simulink model "model_local_observers"  (R2024b)
settings: Solver=ode45  StartTime=0.0  StopTime=150  RelTol=1e-3
values from neighbouring files (symbols this model uses):
  Ad = [ ... (first row only)    [compute_topology_matrices.m]
  G = diag([1 1 1 1 1 1])    [compute_topology_matrices.m]
undefined symbols (not defined in the file or in its folder): A, A_leader, B, C, c, F, K, Lu_obs, noise_free, sigma_followers, sigma_leader, x0, x0_followers, xhat0
settings Model: Creator=siani  LastModifiedBy=siani
settings DebuggingCC: AlgebraicLoopMsg=none

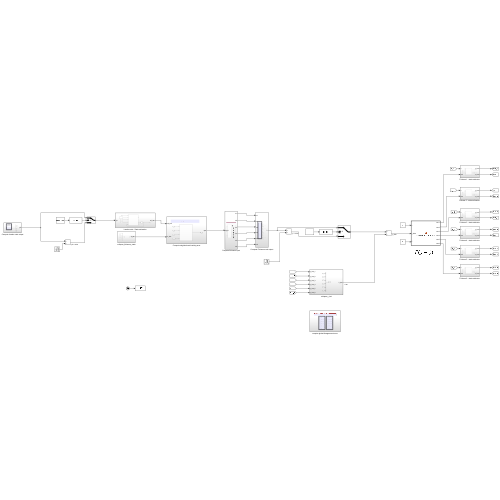
[thumbnail: Simulink's stored preview of the top-level diagram]
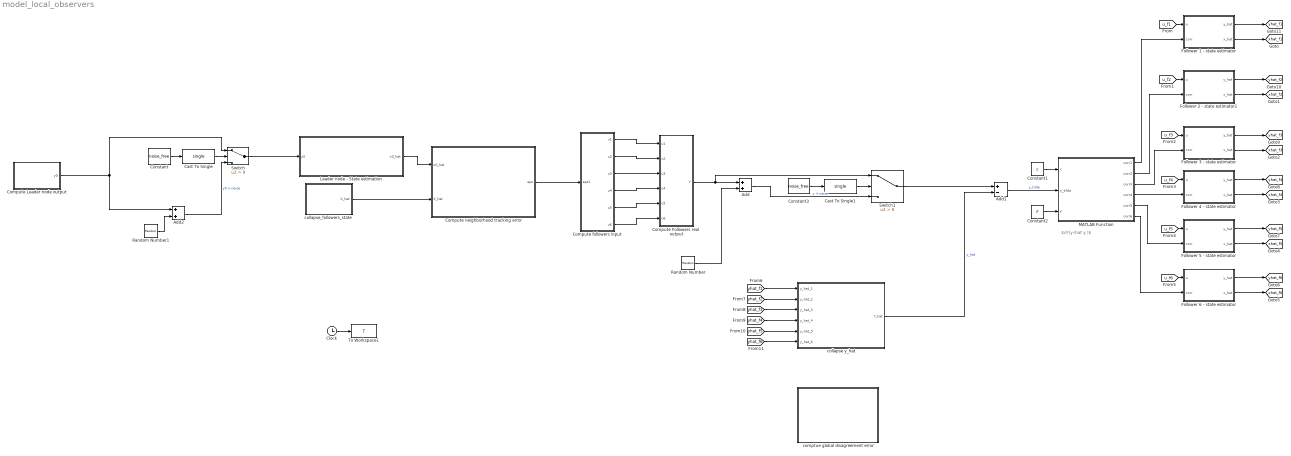
== system model_local_observers ==
  note: $cF(y-\hat y )$
  Add : Sum
  Add1 : Sum  Inputs=+-
  Add2 : Sum
  Cast To Single : DataTypeConversion  OutDataTypeStr=single  SaturateOnIntegerOverflow=off  RndMeth=Floor
  Cast To Single1 : DataTypeConversion  OutDataTypeStr=single  SaturateOnIntegerOverflow=off  RndMeth=Floor
  Clock : Clock
  Compute Followers real output : Subsystem
  Compute Leader node output : Subsystem
  Compute followers input : Subsystem
  Compute neighborhood tracking error : Subsystem
  Constant : Constant  Value=noise_free
  Constant1 : Constant  Value=c
  Constant2 : Constant  Value=F
  Constant3 : Constant  Value=noise_free
  Follower 1 - state estimator : Subsystem
  Follower 2 - state estimator1 : Subsystem
  Follower 3 - state estimator : Subsystem
  Follower 4 - state estimator : Subsystem
  Follower 5 - state estimator : Subsystem
  Follower 6 - state estimator : Subsystem
  Leader node - State estimation : Subsystem
  MATLAB Function : MATLAB Function  TreatAsAtomicUnit=on
  Random Number : RandomNumber  Mean=zeros(6,1)  Variance=sigma_followers^2*ones(6,1)  SampleTime=0.1
  Random Number1 : RandomNumber  Variance=sigma_leader^2  SampleTime=0.1
  Switch : Switch  Criteria=u2 > Threshold  SaturateOnIntegerOverflow=off  InputSameDT=off
  Switch1 : Switch  Criteria=u2 > Threshold  SaturateOnIntegerOverflow=off  InputSameDT=off
  To Workspace1 : ToWorkspace  VariableName=T  SampleTime=-1
  collapse y_hat : Subsystem
  collapse_followers_state : Subsystem
  comptue global disagreement error : Subsystem
  tag scope: xhat_f1=global, xhat_f2=global, xhat_f3=global, xhat_f4=global, xhat_f5=global, xhat_f6=global, yhat_f1=global, yhat_f2=global, yhat_f3=global, yhat_f4=global, yhat_f5=global, yhat_f6=global
  wires:
  Compute Followers real output/1(Y) -> Switch1/1, Add/1
  [u_f1] -> Follower 1 - state estimator/1(u)
  Switch/1 -> Leader node - State estimation/1(y0)
  Switch1/1 -> Add1/1
  Add/1 -> Switch1/3  "y + noise"
  Compute Leader node output/1(y0) -> Add2/1, Switch/1
  collapse y_hat/1(Y_hat) -> Add1/2  "y_hat"
  Add1/1 -> MATLAB Function/2(y_tilda)  "y_tilda"
  [yhat_f1] -> collapse y_hat/1(y_hat_1)
  [yhat_f2] -> collapse y_hat/2(y_hat_2)
  [yhat_f3] -> collapse y_hat/3(y_hat_3)
  [yhat_f4] -> collapse y_hat/4(y_hat_4)
  [yhat_f5] -> collapse y_hat/5(y_hat_5)
  [yhat_f6] -> collapse y_hat/6(y_hat_6)
  Random Number/1 -> Add/2
  Leader node - State estimation/1(x0_hat) -> Compute neighborhood tracking error/1(x0_hat)
  collapse_followers_state/1(X_hat) -> Compute neighborhood tracking error/2(X_hat)
  Constant1/1 -> MATLAB Function/1(c)
  Constant2/1 -> MATLAB Function/3(F)
  MATLAB Function/1(corr1) -> Follower 1 - state estimator/2(corr)
  MATLAB Function/2(corr2) -> Follower 2 - state estimator1/2(corr)
  MATLAB Function/3(corr3) -> Follower 3 - state estimator/2(corr)
  MATLAB Function/4(corr4) -> Follower 4 - state estimator/2(corr)
  MATLAB Function/5(corr5) -> Follower 5 - state estimator/2(corr)
  MATLAB Function/6(corr6) -> Follower 6 - state estimator/2(corr)
  Follower 1 - state estimator/1(y_hat) -> [yhat_f1]
  Follower 1 - state estimator/2(x_hat) -> [xhat_f1]
  Follower 2 - state estimator1/1(y_hat) -> [yhat_f2]
  Follower 2 - state estimator1/2(x_hat) -> [xhat_f2]
  Follower 3 - state estimator/1(y_hat) -> [yhat_f3]
  Follower 3 - state estimator/2(x_hat) -> [xhat_f3]
  Follower 4 - state estimator/1(y_hat) -> [yhat_f4]
  Follower 4 - state estimator/2(x_hat) -> [xhat_f4]
  Follower 5 - state estimator/1(y_hat) -> [yhat_f5]
  Follower 5 - state estimator/2(x_hat) -> [xhat_f5]
  Follower 6 - state estimator/1(y_hat) -> [yhat_f6]
  Follower 6 - state estimator/2(x_hat) -> [xhat_f6]
  [u_f2] -> Follower 2 - state estimator1/1(u)
  [u_f3] -> Follower 3 - state estimator/1(u)
  [u_f4] -> Follower 4 - state estimator/1(u)
  [u_f5] -> Follower 5 - state estimator/1(u)
  [u_f6] -> Follower 6 - state estimator/1(u)
  Constant3/1 -> Cast To Single1/1
  Cast To Single1/1 -> Switch1/2
  Add2/1 -> Switch/3  "y0 + noise"
  Cast To Single/1 -> Switch/2
  Constant/1 -> Cast To Single/1
  Random Number1/1 -> Add2/2
  Clock/1 -> To Workspace1/1
  Compute neighborhood tracking error/1(eps) -> Compute followers input/1(eps1)
  Compute followers input/1(u1) -> Compute Followers real output/1(u1)
  Compute followers input/2(u2) -> Compute Followers real output/2(u2)
  Compute followers input/3(u3) -> Compute Followers real output/3(u3)
  Compute followers input/4(u4) -> Compute Followers real output/4(u4)
  Compute followers input/5(u5) -> Compute Followers real output/5(u5)
  Compute followers input/6(u6) -> Compute Followers real output/6(u6)

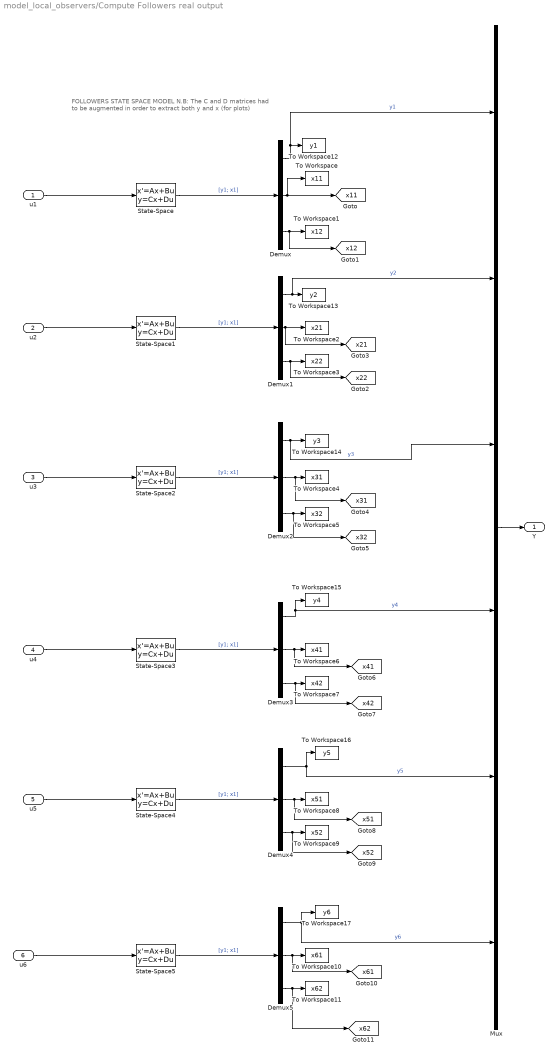
== system model_local_observers/Compute Followers real output ==
  note: FOLLOWERS STATE SPACE MODEL
      |
      | N.B: The C and D matrices had to be augmented in order to extract both y and x (for plots)
  u1 : Inport
  u2 : Inport  Port=2
  u3 : Inport  Port=3
  u4 : Inport  Port=4
  u5 : Inport  Port=5
  u6 : Inport  Port=6
  Demux{,1..5} (6 alike) : Demux  Outputs=[1 1 1]
  Mux : Mux  Inputs=[1 1 1 1 1 1]
  State-Space{,1..5} (6 alike) : StateSpace  A=A  B=B  C=[C;eye(2)]  D=[0;0;0]  InitialCondition=x0_followers
  To Workspace : ToWorkspace  VariableName=x11  SampleTime=-1
  To Workspace1 : ToWorkspace  VariableName=x12  SampleTime=-1
  To Workspace10 : ToWorkspace  VariableName=x61  SampleTime=-1
  To Workspace11 : ToWorkspace  VariableName=x62  SampleTime=-1
  To Workspace12 : ToWorkspace  VariableName=y1  SampleTime=-1
  To Workspace13 : ToWorkspace  VariableName=y2  SampleTime=-1
  To Workspace14 : ToWorkspace  VariableName=y3  SampleTime=-1
  To Workspace15 : ToWorkspace  VariableName=y4  SampleTime=-1
  To Workspace16 : ToWorkspace  VariableName=y5  SampleTime=-1
  To Workspace17 : ToWorkspace  VariableName=y6  SampleTime=-1
  To Workspace2 : ToWorkspace  VariableName=x21  SampleTime=-1
  To Workspace3 : ToWorkspace  VariableName=x22  SampleTime=-1
  To Workspace4 : ToWorkspace  VariableName=x31  SampleTime=-1
  To Workspace5 : ToWorkspace  VariableName=x32  SampleTime=-1
  To Workspace6 : ToWorkspace  VariableName=x41  SampleTime=-1
  To Workspace7 : ToWorkspace  VariableName=x42  SampleTime=-1
  To Workspace8 : ToWorkspace  VariableName=x51  SampleTime=-1
  To Workspace9 : ToWorkspace  VariableName=x52  SampleTime=-1
  Y : Outport
  tag scope: x11=global, x12=global, x21=global, x22=global, x31=global, x32=global, x41=global, x42=global, x51=global, x52=global, x61=global, x62=global
  wires:
  u1/1 -> State-Space/1
  Mux/1 -> Y/1
  State-Space/1 -> Demux/1  "[y1; x1]"
  Demux/1 -> To Workspace12/1, Mux/1  "y1"
  Demux/2 -> To Workspace/1, [x11]
  Demux/3 -> [x12], To Workspace1/1
  Demux1/2 -> [x21], To Workspace2/1
  State-Space1/1 -> Demux1/1  "[y1; x1]"
  Demux1/3 -> [x22], To Workspace3/1
  Demux1/1 -> Mux/2, To Workspace13/1  "y2"
  u2/1 -> State-Space1/1
  Demux2/1 -> Mux/3, To Workspace14/1  "y3"
  Demux2/3 -> [x32], To Workspace5/1
  Demux2/2 -> [x31], To Workspace4/1
  State-Space2/1 -> Demux2/1  "[y1; x1]"
  u3/1 -> State-Space2/1
  Demux3/2 -> [x41], To Workspace6/1
  Demux3/3 -> [x42], To Workspace7/1
  State-Space3/1 -> Demux3/1  "[y1; x1]"
  Demux3/1 -> To Workspace15/1, Mux/4  "y4"
  u4/1 -> State-Space3/1
  Demux4/3 -> [x52], To Workspace9/1
  Demux4/2 -> [x51], To Workspace8/1
  State-Space4/1 -> Demux4/1  "[y1; x1]"
  u5/1 -> State-Space4/1
  State-Space5/1 -> Demux5/1  "[y1; x1]"
  Demux5/2 -> [x61], To Workspace10/1
  Demux5/3 -> [x62], To Workspace11/1
  u6/1 -> State-Space5/1
  Demux4/1 -> Mux/5, To Workspace16/1  "y5"
  Demux5/1 -> Mux/6, To Workspace17/1  "y6"

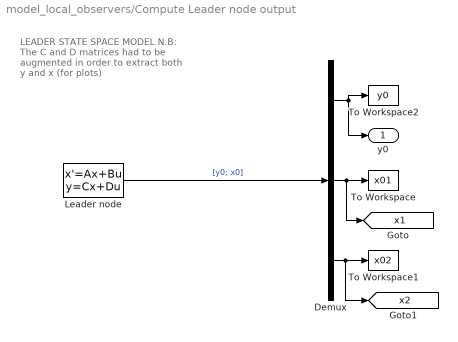
== system model_local_observers/Compute Leader node output ==
  note: LEADER STATE SPACE MODEL
      |
      | N.B: The C and D matrices had to be augmented in order to extract both y and x (for plots)
  Demux : Demux  Outputs=[1 1 1]
  Leader node : StateSpace  A=A_leader  B=[0 0]'  C=[C;eye(2)]  D=[0;0;0]  InitialCondition=x0
  To Workspace : ToWorkspace  VariableName=x01  SampleTime=-1
  To Workspace1 : ToWorkspace  VariableName=x02  SampleTime=-1
  To Workspace2 : ToWorkspace  VariableName=y0  SampleTime=-1
  y0 : Outport
  tag scope: x1=global, x2=global
  wires:
  Leader node/1 -> Demux/1  "[y0; x0]"
  Demux/1 -> To Workspace2/1, y0/1
  Demux/2 -> [x1], To Workspace/1
  Demux/3 -> [x2], To Workspace1/1

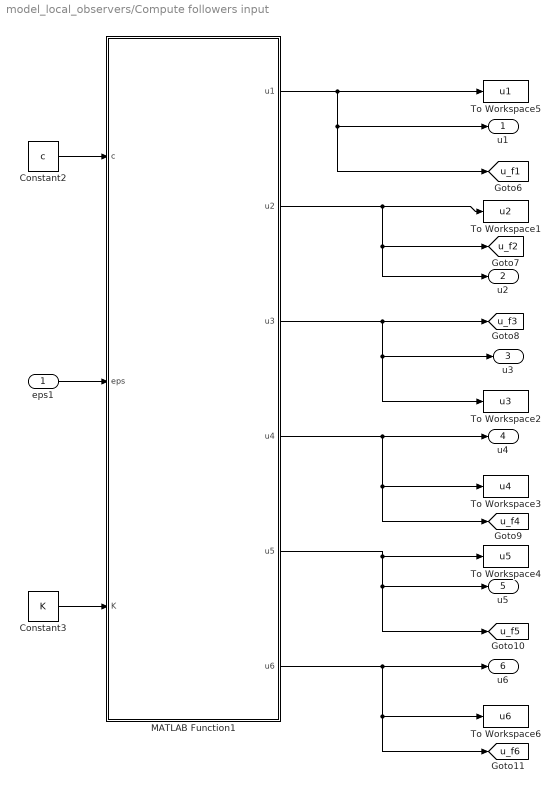
== system model_local_observers/Compute followers input ==
  eps1 : Inport
  Constant2 : Constant  Value=c
  Constant3 : Constant  Value=K  VectorParams1D=off
  MATLAB Function1 : MATLAB Function  TreatAsAtomicUnit=on
  To Workspace1 : ToWorkspace  VariableName=u2  SampleTime=-1
  To Workspace2 : ToWorkspace  VariableName=u3  SampleTime=-1
  To Workspace3 : ToWorkspace  VariableName=u4  SampleTime=-1
  To Workspace4 : ToWorkspace  VariableName=u5  SampleTime=-1
  To Workspace5 : ToWorkspace  VariableName=u1  SampleTime=-1
  To Workspace6 : ToWorkspace  VariableName=u6  SampleTime=-1
  u1 : Outport
  u2 : Outport  Port=2
  u3 : Outport  Port=3
  u4 : Outport  Port=4
  u5 : Outport  Port=5
  u6 : Outport  Port=6
  tag scope: u_f1=global, u_f2=global, u_f3=global, u_f4=global, u_f5=global, u_f6=global
  wires:
  MATLAB Function1/3(u3) -> u3/1, To Workspace2/1, [u_f3]
  MATLAB Function1/5(u5) -> u5/1, [u_f5], To Workspace4/1
  MATLAB Function1/6(u6) -> [u_f6], To Workspace6/1, u6/1
  eps1/1 -> MATLAB Function1/2(eps)
  MATLAB Function1/4(u4) -> [u_f4], To Workspace3/1, u4/1
  Constant2/1 -> MATLAB Function1/1(c)
  Constant3/1 -> MATLAB Function1/3(K)
  MATLAB Function1/2(u2) -> u2/1, [u_f2], To Workspace1/1
  MATLAB Function1/1(u1) -> u1/1, [u_f1], To Workspace5/1

== system model_local_observers/Compute neighborhood tracking error ==
  x0_hat : Inport
  X_hat : Inport  Port=2
  Constant : Constant  Value=Ad
  Constant1 : Constant  Value=G
  MATLAB Function : MATLAB Function  TreatAsAtomicUnit=on
  eps : Outport
  wires:
  x0_hat/1 -> MATLAB Function/2(x0_hat)
  Constant/1 -> MATLAB Function/3(Ad)
  Constant1/1 -> MATLAB Function/4(G)
  X_hat/1 -> MATLAB Function/1(x_hat)
  MATLAB Function/1(eps) -> eps/1

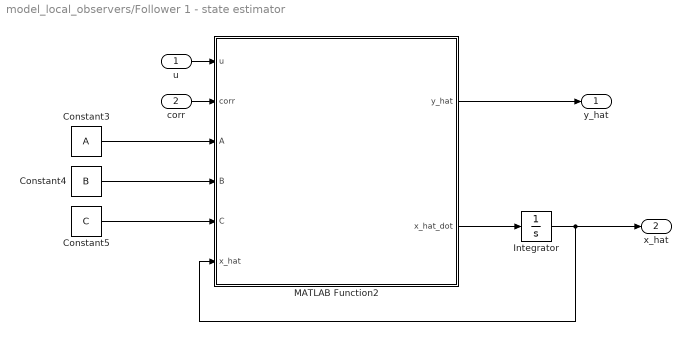
== system model_local_observers/Follower 1 - state estimator ==
  u : Inport
  corr : Inport  Port=2
  Constant3 : Constant  Value=A
  Constant4 : Constant  Value=B  VectorParams1D=off
  Constant5 : Constant  Value=C  VectorParams1D=off
  Integrator : Integrator  InitialCondition=xhat0
  MATLAB Function2 : MATLAB Function  TreatAsAtomicUnit=on
  y_hat : Outport
  x_hat : Outport  Port=2
  wires:
  MATLAB Function2/1(y_hat) -> y_hat/1
  corr/1 -> MATLAB Function2/2(corr)
  MATLAB Function2/2(x_hat_dot) -> Integrator/1
  Integrator/1 -> MATLAB Function2/6(x_hat), x_hat/1
  Constant3/1 -> MATLAB Function2/3(A)
  u/1 -> MATLAB Function2/1(u)
  Constant4/1 -> MATLAB Function2/4(B)
  Constant5/1 -> MATLAB Function2/5(C)

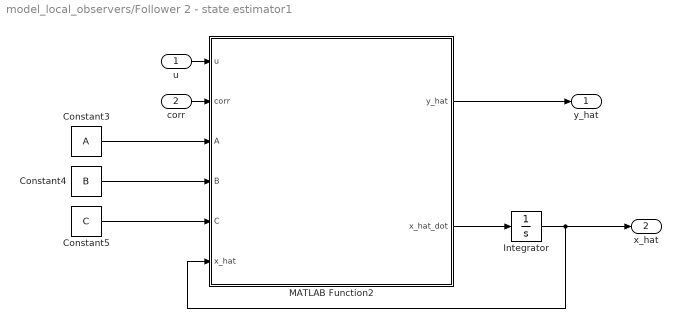
== system model_local_observers/Follower 2 - state estimator1 ==
  u : Inport
  corr : Inport  Port=2
  Constant3 : Constant  Value=A
  Constant4 : Constant  Value=B  VectorParams1D=off
  Constant5 : Constant  Value=C  VectorParams1D=off
  Integrator : Integrator  InitialCondition=xhat0
  MATLAB Function2 : MATLAB Function  TreatAsAtomicUnit=on
  y_hat : Outport
  x_hat : Outport  Port=2
  wires:
  Constant5/1 -> MATLAB Function2/5(C)
  Constant4/1 -> MATLAB Function2/4(B)
  u/1 -> MATLAB Function2/1(u)
  Constant3/1 -> MATLAB Function2/3(A)
  Integrator/1 -> MATLAB Function2/6(x_hat), x_hat/1
  MATLAB Function2/2(x_hat_dot) -> Integrator/1
  corr/1 -> MATLAB Function2/2(corr)
  MATLAB Function2/1(y_hat) -> y_hat/1

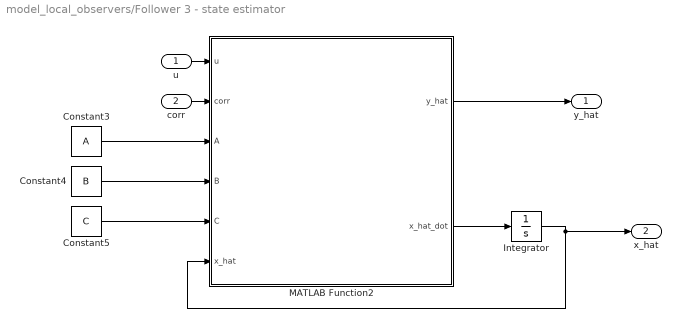
== system model_local_observers/Follower 3 - state estimator ==
  u : Inport
  corr : Inport  Port=2
  Constant3 : Constant  Value=A
  Constant4 : Constant  Value=B  VectorParams1D=off
  Constant5 : Constant  Value=C  VectorParams1D=off
  Integrator : Integrator  InitialCondition=xhat0
  MATLAB Function2 : MATLAB Function  TreatAsAtomicUnit=on
  y_hat : Outport
  x_hat : Outport  Port=2
  wires:
  MATLAB Function2/1(y_hat) -> y_hat/1
  corr/1 -> MATLAB Function2/2(corr)
  MATLAB Function2/2(x_hat_dot) -> Integrator/1
  Integrator/1 -> MATLAB Function2/6(x_hat), x_hat/1
  Constant3/1 -> MATLAB Function2/3(A)
  u/1 -> MATLAB Function2/1(u)
  Constant4/1 -> MATLAB Function2/4(B)
  Constant5/1 -> MATLAB Function2/5(C)

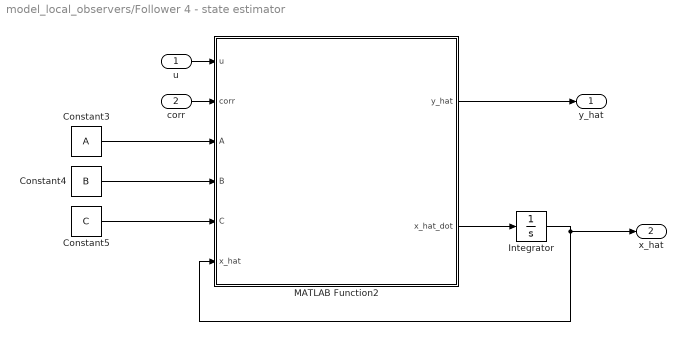
== system model_local_observers/Follower 4 - state estimator ==
  u : Inport
  corr : Inport  Port=2
  Constant3 : Constant  Value=A
  Constant4 : Constant  Value=B  VectorParams1D=off
  Constant5 : Constant  Value=C  VectorParams1D=off
  Integrator : Integrator  InitialCondition=xhat0
  MATLAB Function2 : MATLAB Function  TreatAsAtomicUnit=on
  y_hat : Outport
  x_hat : Outport  Port=2
  wires:
  Constant5/1 -> MATLAB Function2/5(C)
  Constant4/1 -> MATLAB Function2/4(B)
  u/1 -> MATLAB Function2/1(u)
  Constant3/1 -> MATLAB Function2/3(A)
  Integrator/1 -> MATLAB Function2/6(x_hat), x_hat/1
  MATLAB Function2/2(x_hat_dot) -> Integrator/1
  corr/1 -> MATLAB Function2/2(corr)
  MATLAB Function2/1(y_hat) -> y_hat/1

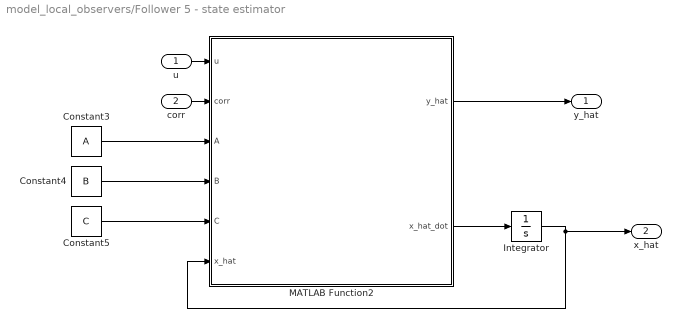
== system model_local_observers/Follower 5 - state estimator ==
  u : Inport
  corr : Inport  Port=2
  Constant3 : Constant  Value=A
  Constant4 : Constant  Value=B  VectorParams1D=off
  Constant5 : Constant  Value=C  VectorParams1D=off
  Integrator : Integrator  InitialCondition=xhat0
  MATLAB Function2 : MATLAB Function  TreatAsAtomicUnit=on
  y_hat : Outport
  x_hat : Outport  Port=2
  wires:
  MATLAB Function2/1(y_hat) -> y_hat/1
  corr/1 -> MATLAB Function2/2(corr)
  MATLAB Function2/2(x_hat_dot) -> Integrator/1
  Integrator/1 -> MATLAB Function2/6(x_hat), x_hat/1
  Constant3/1 -> MATLAB Function2/3(A)
  u/1 -> MATLAB Function2/1(u)
  Constant4/1 -> MATLAB Function2/4(B)
  Constant5/1 -> MATLAB Function2/5(C)

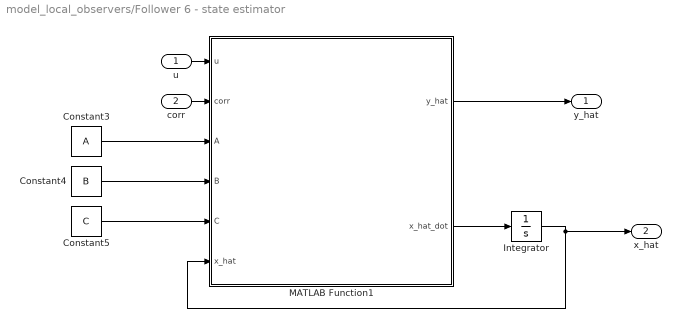
== system model_local_observers/Follower 6 - state estimator ==
  u : Inport
  corr : Inport  Port=2
  Constant3 : Constant  Value=A
  Constant4 : Constant  Value=B  VectorParams1D=off
  Constant5 : Constant  Value=C  VectorParams1D=off
  Integrator : Integrator  InitialCondition=xhat0
  MATLAB Function1 : MATLAB Function  TreatAsAtomicUnit=on
  y_hat : Outport
  x_hat : Outport  Port=2
  wires:
  Constant5/1 -> MATLAB Function1/5(C)
  Constant4/1 -> MATLAB Function1/4(B)
  u/1 -> MATLAB Function1/1(u)
  Constant3/1 -> MATLAB Function1/3(A)
  Integrator/1 -> MATLAB Function1/6(x_hat), x_hat/1
  MATLAB Function1/2(x_hat_dot) -> Integrator/1
  corr/1 -> MATLAB Function1/2(corr)
  MATLAB Function1/1(y_hat) -> y_hat/1

== system model_local_observers/Leader node - State estimation ==
  y0 : Inport
  Constant3 : Constant  Value=A_leader
  Constant4 : Constant  Value=Lu_obs  VectorParams1D=off
  Constant5 : Constant  Value=C  VectorParams1D=off
  Integrator : Integrator  InitialCondition=xhat0
  MATLAB Function1 : MATLAB Function  TreatAsAtomicUnit=on
  x0_hat : Outport
  wires:
  Constant3/1 -> MATLAB Function1/2(A)
  Integrator/1 -> MATLAB Function1/5(x0_hat), x0_hat/1
  Constant5/1 -> MATLAB Function1/3(C)
  Constant4/1 -> MATLAB Function1/4(L)
  MATLAB Function1/2(x0_hat_dot) -> Integrator/1
  y0/1 -> MATLAB Function1/1(y0)

== system model_local_observers/collapse y_hat ==
  y_hat_1 : Inport
  y_hat_2 : Inport  Port=2
  y_hat_3 : Inport  Port=3
  y_hat_4 : Inport  Port=4
  y_hat_5 : Inport  Port=5
  y_hat_6 : Inport  Port=6
  Mux : Mux  Inputs=6
  Y_hat : Outport
  wires:
  y_hat_1/1 -> Mux/1
  Mux/1 -> Y_hat/1
  y_hat_4/1 -> Mux/4
  y_hat_3/1 -> Mux/3
  y_hat_6/1 -> Mux/6
  y_hat_2/1 -> Mux/2
  y_hat_5/1 -> Mux/5

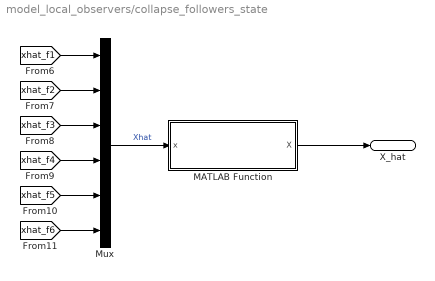
== system model_local_observers/collapse_followers_state ==
  MATLAB Function : MATLAB Function  TreatAsAtomicUnit=on
  Mux : Mux  Inputs=[2 2 2 2 2 2 ]
  X_hat : Outport
  wires:
  [xhat_f2] -> Mux/2
  [xhat_f5] -> Mux/5
  [xhat_f6] -> Mux/6
  [xhat_f3] -> Mux/3
  [xhat_f4] -> Mux/4
  [xhat_f1] -> Mux/1
  MATLAB Function/1(X) -> X_hat/1
  Mux/1 -> MATLAB Function/1(x)  "Xhat"

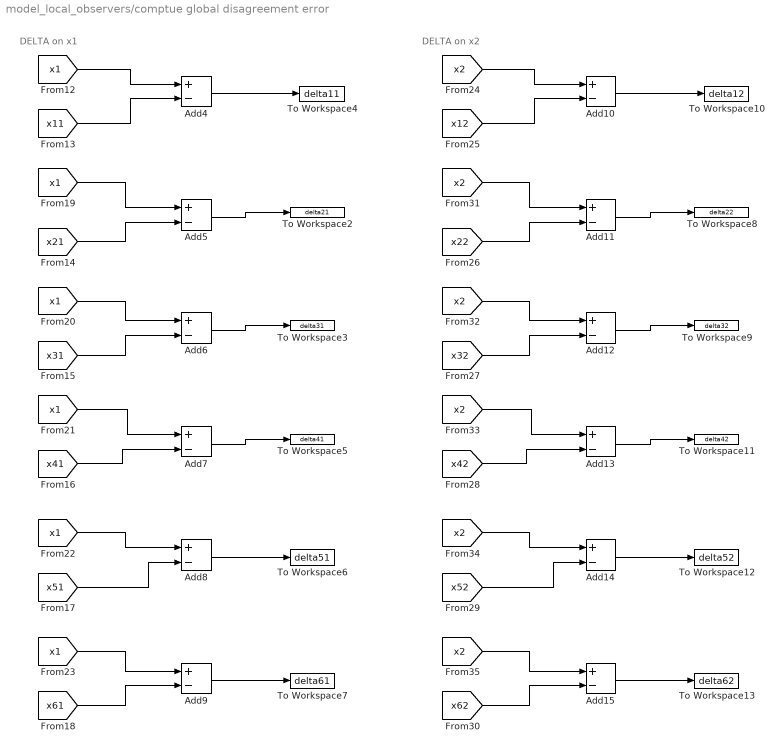
== system model_local_observers/comptue global disagreement error ==
  note: DELTA on x2
  note: DELTA on x1
  Add{4..15} (12 alike) : Sum  Inputs=+-
  To Workspace10 : ToWorkspace  VariableName=delta12  SampleTime=-1
  To Workspace11 : ToWorkspace  VariableName=delta42  SampleTime=-1
  To Workspace12 : ToWorkspace  VariableName=delta52  SampleTime=-1
  To Workspace13 : ToWorkspace  VariableName=delta62  SampleTime=-1
  To Workspace2 : ToWorkspace  VariableName=delta21  SampleTime=-1
  To Workspace3 : ToWorkspace  VariableName=delta31  SampleTime=-1
  To Workspace4 : ToWorkspace  VariableName=delta11  SampleTime=-1
  To Workspace5 : ToWorkspace  VariableName=delta41  SampleTime=-1
  To Workspace6 : ToWorkspace  VariableName=delta51  SampleTime=-1
  To Workspace7 : ToWorkspace  VariableName=delta61  SampleTime=-1
  To Workspace8 : ToWorkspace  VariableName=delta22  SampleTime=-1
  To Workspace9 : ToWorkspace  VariableName=delta32  SampleTime=-1
  wires:
  Add14/1 -> To Workspace12/1
  [x62] -> Add15/2
  Add8/1 -> To Workspace6/1
  Add11/1 -> To Workspace8/1
  Add12/1 -> To Workspace9/1
  [x2] -> Add13/1
  Add10/1 -> To Workspace10/1
  Add13/1 -> To Workspace11/1
  Add4/1 -> To Workspace4/1
  [x52] -> Add14/2
  Add6/1 -> To Workspace3/1
  [x12] -> Add10/2
  [x2] -> Add10/1
  Add5/1 -> To Workspace2/1
  [x51] -> Add8/2
  Add15/1 -> To Workspace13/1
  [x2] -> Add12/1
  Add9/1 -> To Workspace7/1
  [x1] -> Add8/1
  [x2] -> Add14/1
  [x2] -> Add15/1
  [x41] -> Add7/2
  [x1] -> Add6/1
  [x32] -> Add12/2
  [x22] -> Add11/2
  [x42] -> Add13/2
  [x11] -> Add4/2
  [x2] -> Add11/1
  [x21] -> Add5/2
  [x31] -> Add6/2
  [x1] -> Add5/1
  [x61] -> Add9/2
  [x1] -> Add9/1
  [x1] -> Add4/1
  [x1] -> Add7/1
  Add7/1 -> To Workspace5/1

== matlab function model_local_observers/Follower 4 - state estimator/MATLAB Function2 ==
  data: y_hat output; u input; corr input; x_hat_dot output; A input; B input; C input; x_hat input

function [y_hat, x_hat_dot] = compute_follower_state_estimation(u, corr, A, B, C, x_hat)
    
    y_hat = 0;
    x_hat_dot = zeros(2,1);

    
    x_hat_dot = A*x_hat + B*u - corr;
    y_hat = C*x_hat;
end

== matlab function model_local_observers/Follower 6 - state estimator/MATLAB Function1 ==
  data: y_hat output; u input; corr input; x_hat_dot output; A input; B input; C input; x_hat input

function [y_hat, x_hat_dot] = compute_follower_state_estimation(u, corr, A, B, C, x_hat)
    
    y_hat = 0;
    x_hat_dot = zeros(2,1);

    
    x_hat_dot = A*x_hat + B*u - corr;
    y_hat = C*x_hat;
end

== matlab function model_local_observers/Leader node - State estimation/MATLAB Function1 ==
  data: y0 input; y0_hat output; A input; C input; L input; x0_hat input; x0_hat_dot output
% Luenberger estimator for Leader state
function [y0_hat, x0_hat_dot] = compute_leader_estimation(y0, A, C, L, x0_hat)
    x0_hat_dot= zeros(2,1);
    y0_hat = 0;

    x0_hat_dot = (A - L*C)*x0_hat + L*y0;
end

== matlab function model_local_observers/Follower 5 - state estimator/MATLAB Function2 ==
  data: y_hat output; u input; corr input; x_hat_dot output; A input; B input; C input; x_hat input

function [y_hat, x_hat_dot] = compute_follower_state_estimation(u, corr, A, B, C, x_hat)
    
    y_hat = 0;
    x_hat_dot = zeros(2,1);

    
    x_hat_dot = A*x_hat + B*u - corr;
    y_hat = C*x_hat;
end

== matlab function model_local_observers/Compute neighborhood tracking error/MATLAB Function ==
  data: x_hat input; eps output; x0_hat input; Ad input; G input

% COMPUTE_NEIGH_TRACKING_ERROR Computes the neighborhood tracking error
%   Inputs:
%       x_hat  - (n x N) Matrix of estimated states for all N agents.
%               Taken as input
%       x0_hat - (n x 1) Vector of the leader's estimated state (target trajectory).
%               Taken as input
%
%       Ad     - (N x N) Adjacency matrix of the communication graph. 
%               Taken as input
%
%       G      - (N x N) Pinning gain matrix (typically diagonal). 
%                Taken as input
%


function eps = compute_neigh_tracking_error(x_hat, x0_hat, Ad, G)
    n = 2;
    N= 6;
    eps = zeros(n, N);

    for i=1:N
        tracking_error = zeros(n, 1);
    
        for j = 1:N
            tracking_error = tracking_error + Ad(i,j)*(x_hat(:,j)-x_hat(:,i));
        end
        
        tracking_error = tracking_error + G(i,i)*(x0_hat - x_hat(:,i));
        eps(:,i) = tracking_error;
    
    end
end

== matlab function model_local_observers/Compute followers input/MATLAB Function1 ==
  data: c input; u1 output; eps input; K input; u2 output; u3 output; u4 output; u5 output; u6 output
function [u1, u2, u3, u4, u5, u6] = compute_ui(c, eps, K)
    u1 = 0;
    u2 = 0;
    u3 = 0;
    u4 = 0;
    u5 = 0;
    u6 = 0;

    u1 = c*K*eps(:, 1);
    u2 = c*K*eps(:, 2);
    u3 = c*K*eps(:, 3);
    u4 = c*K*eps(:, 4);
    u5 = c*K*eps(:, 5);
    u6 = c*K*eps(:, 6);
end

== matlab function model_local_observers/MATLAB Function ==
  data: c input; corr1 output; y_tilda input; F input; corr2 output; corr3 output; corr4 output; corr5 output; corr6 output
function [corr1, corr2, corr3, corr4, corr5, corr6] = compute_obs_correction(c, y_tilda, F)
    corr1 = c*F*y_tilda(1);
    corr2 = c*F*y_tilda(2);
    corr3 = c*F*y_tilda(3);
    corr4 = c*F*y_tilda(4);
    corr5 = c*F*y_tilda(5);
    corr6 = c*F*y_tilda(6);
end

== matlab function model_local_observers/collapse_followers_state/MATLAB Function ==
  data: x input; X output
function X = reshape_to_matrix(x)

X = reshape(x,2,6);

== matlab function model_local_observers/Follower 1 - state estimator/MATLAB Function2 ==
  data: y_hat output; u input; corr input; x_hat_dot output; A input; B input; C input; x_hat input

function [y_hat, x_hat_dot] = compute_follower_state_estimation(u, corr, A, B, C, x_hat)
    
    y_hat = 0;
    x_hat_dot = zeros(2,1);

    
    x_hat_dot = A*x_hat + B*u - corr;
    y_hat = C*x_hat;
end

== matlab function model_local_observers/Follower 2 - state estimator1/MATLAB Function2 ==
  data: y_hat output; u input; corr input; x_hat_dot output; A input; B input; C input; x_hat input

function [y_hat, x_hat_dot] = compute_follower_state_estimation(u, corr, A, B, C, x_hat)
    
    y_hat = 0;
    x_hat_dot = zeros(2,1);

    
    x_hat_dot = A*x_hat + B*u - corr;
    y_hat = C*x_hat;
end

== matlab function model_local_observers/Follower 3 - state estimator/MATLAB Function2 ==
  data: y_hat output; u input; corr input; x_hat_dot output; A input; B input; C input; x_hat input

function [y_hat, x_hat_dot] = compute_follower_state_estimation(u, corr, A, B, C, x_hat)
    
    y_hat = 0;
    x_hat_dot = zeros(2,1);

    
    x_hat_dot = A*x_hat + B*u - corr;
    y_hat = C*x_hat;
end
